simulink model "untitled"  (R2022a)
settings: Solver=VariableStepAuto  StartTime=0.0  StopTime=6  RelTol=1e-3
libraries: spsSeriesRLCBranchLib x8, spsDiodeLib x6, spsVoltageMeasurementLib x4, spsACVoltageSourceLib x3, spsGroundLib x3, spsCurrentMeasurementLib x1, spsPermanentMagnetSynchronousMachineLib x1, spsThreePhaseVIMeasurementLib x1
settings Model: Creator=glopezc  LastModifiedBy=glopezc

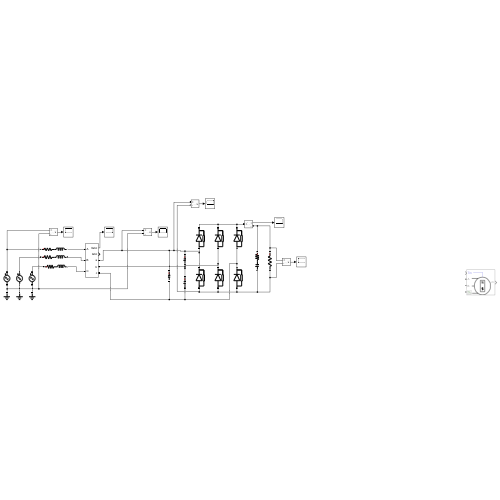
[thumbnail: Simulink's stored preview of the top-level diagram]
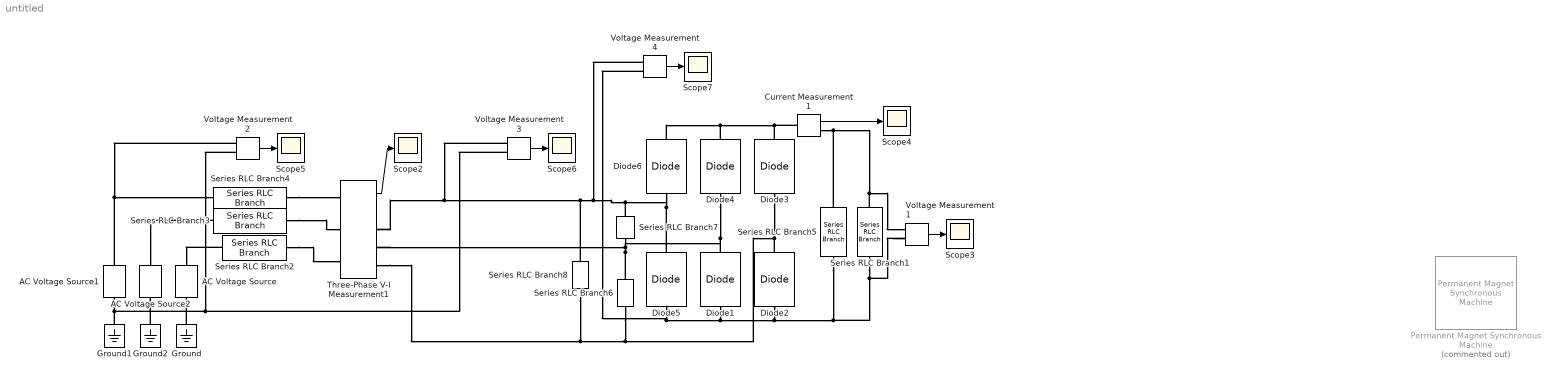
== system untitled ==
  AC Voltage Source : spsACVoltageSourceLib/AC Voltage Source  Amplitude=453  Phase=-120  Frequency=46  SampleTime=0  Measurements=None  BusType=swing  Pref=10e3  Qref=0  Qmin=-inf  Qmax=+inf
  AC Voltage Source1 : spsACVoltageSourceLib/AC Voltage Source  Amplitude=453  Phase=0  Frequency=46  SampleTime=0  Measurements=None  BusType=swing  Pref=10e3  Qref=0  Qmin=-inf  Qmax=+inf
  AC Voltage Source2 : spsACVoltageSourceLib/AC Voltage Source  Amplitude=453  Phase=120  Frequency=46  SampleTime=0  Measurements=None  BusType=swing  Pref=10e3  Qref=0  Qmin=-inf  Qmax=+inf
  Current Measurement1 : spsCurrentMeasurementLib/Current Measurement  PhasorSimulation=off  OutputType=Complex  PSBequivalent=0
  Diode{1..6} (6 alike) : spsDiodeLib/Diode  Ron=0.01  Lon=0  Vf=0.6  IC=0  UseSnubber=0  Rs=500  Cs=250e-9  Measurements=off
  Ground : spsGroundLib/Ground  LConnTagsString=a
  Ground1 : spsGroundLib/Ground  LConnTagsString=a
  Ground2 : spsGroundLib/Ground  LConnTagsString=a
  Permanent Magnet Synchronous Machine : spsPermanentMagnetSynchronousMachineLib/Permanent Magnet Synchronous Machine  Commented=on  NbPhases=3  FluxDistribution=Sinusoidal  RotorType=Round  MechanicalLoad=Torque Tm  PresetModel=No  ShowDetailedParameters=on  MeasurementBus=off  Resistance=0.0485  Inductance=8.5e-3  dqInductances=[8.5e-3,8.5e-3]  La=0.000395  MachineConstant=Flux linkage established by magnets (V.s)  Flux=0.1194  VoltageCst=86.6271  TorqueCst=0.7164  Flat=120  Mechanical=[0.0027 0.0004924 4 0]  PolePairs=4  InitialConditions=[0,0, 0,0]  InitialConditions5ph=[0 0 0 0 0 0]  RefAngle=90 degrees behind phase A axis (modified Park)  IterativeDiscreteModel=Trapezoidal non iterative  TsBlock=-1  TsPowergui=0
  Scope{2..7} (6 alike) : Scope
  Series RLC Branch1 : spsSeriesRLCBranchLib/Series RLC Branch  LConnTagsString=__new0  RConnTagsString=__new0  BranchType=R  Resistance=.022e3  Inductance=1e-3  SetiL0=off  InitialCurrent=0  Capacitance=1e-6  Setx0=off  InitialVoltage=0  Measurements=None
  Series RLC Branch2 : spsSeriesRLCBranchLib/Series RLC Branch  LConnTagsString=__new0  RConnTagsString=__new0  BranchType=RL  Resistance=.51  Inductance=12.8e-3  SetiL0=off  InitialCurrent=0  Capacitance=1e-6  Setx0=off  InitialVoltage=0  Measurements=None
  Series RLC Branch3 : spsSeriesRLCBranchLib/Series RLC Branch  LConnTagsString=__new0  RConnTagsString=__new0  BranchType=RL  Resistance=.51  Inductance=12.8e-3  SetiL0=off  InitialCurrent=0  Capacitance=1e-6  Setx0=off  InitialVoltage=0  Measurements=None
  Series RLC Branch4 : spsSeriesRLCBranchLib/Series RLC Branch  LConnTagsString=__new0  RConnTagsString=__new0  BranchType=RL  Resistance=.51  Inductance=12.8e-3  SetiL0=off  InitialCurrent=0  Capacitance=1e-6  Setx0=off  InitialVoltage=0  Measurements=None
  Series RLC Branch5 : spsSeriesRLCBranchLib/Series RLC Branch  LConnTagsString=__new0  RConnTagsString=__new0  BranchType=RC  Resistance=.00084  Inductance=1e-3  SetiL0=off  InitialCurrent=0  Capacitance=2200e-6  Setx0=off  InitialVoltage=0  Measurements=None
  Series RLC Branch6 : spsSeriesRLCBranchLib/Series RLC Branch  LConnTagsString=__new0  RConnTagsString=__new0  BranchType=C  Resistance=0.001  Inductance=1e-3  SetiL0=off  InitialCurrent=0  Capacitance=55e-6  Setx0=off  InitialVoltage=0  Measurements=None
  Series RLC Branch7 : spsSeriesRLCBranchLib/Series RLC Branch  LConnTagsString=__new0  RConnTagsString=__new0  BranchType=C  Resistance=0.001  Inductance=1e-3  SetiL0=off  InitialCurrent=0  Capacitance=55e-6  Setx0=off  InitialVoltage=0  Measurements=None
  Series RLC Branch8 : spsSeriesRLCBranchLib/Series RLC Branch  LConnTagsString=__new0  RConnTagsString=__new0  BranchType=C  Resistance=0.001  Inductance=1e-3  SetiL0=off  InitialCurrent=0  Capacitance=55e-6  Setx0=off  InitialVoltage=0  Measurements=None
  Three-Phase V-I Measurement1 : spsThreePhaseVIMeasurementLib/Three-Phase V-I Measurement  VoltageMeasurement=phase-to-ground  SetLabelV=off  LabelV=Vabc  Vpu=off  VpuLL=off  CurrentMeasurement=yes  SetLabelI=off  LabelI=Iabc  Ipu=off  Pbase=100e6  Vbase=500e3  OutputType=Complex  PhasorSimulation=off  PSBequivalent=0
  Voltage Measurement{1..4} (4 alike) : spsVoltageMeasurementLib/Voltage Measurement  PhasorSimulation=off  OutputType=Complex  PSBequivalent=0
  wires:
  Current Measurement1/1 -> Scope4/1
  Voltage Measurement1/1 -> Scope3/1
  Three-Phase V-I Measurement1/1 -> Scope2/1
  Voltage Measurement2/1 -> Scope5/1
  Voltage Measurement3/1 -> Scope6/1
  Voltage Measurement4/1 -> Scope7/1
  connections:
  Three-Phase V-I Measurement1/RConn3 -- Series RLC Branch6/RConn1 -- Diode3/LConn1 -- Diode2/RConn1 -- Series RLC Branch8/RConn1
  Series RLC Branch7/RConn1 -- Three-Phase V-I Measurement1/RConn2 -- Diode4/LConn1 -- Diode1/RConn1 -- Series RLC Branch6/LConn1
  Current Measurement1/LConn1 -- Diode3/RConn1 -- Diode6/RConn1 -- Diode4/RConn1
  Voltage Measurement3/LConn1 -- Three-Phase V-I Measurement1/RConn1 -- Series RLC Branch8/LConn1 -- Series RLC Branch7/LConn1 -- Diode5/RConn1 -- Diode6/LConn1 -- Voltage Measurement4/LConn1
  Ground2/LConn1 -- AC Voltage Source2/LConn1
  Ground/LConn1 -- AC Voltage Source/LConn1
  Ground1/LConn1 -- Voltage Measurement2/LConn2 -- Voltage Measurement3/LConn2 -- AC Voltage Source1/LConn1
  Series RLC Branch1/RConn1 -- Voltage Measurement4/LConn2 -- Diode5/LConn1 -- Diode1/LConn1 -- Diode2/LConn1 -- Series RLC Branch5/RConn1 -- Voltage Measurement1/LConn2
  Series RLC Branch1/LConn1 -- Series RLC Branch5/LConn1 -- Current Measurement1/RConn1 -- Voltage Measurement1/LConn1
  Series RLC Branch2/RConn1 -- Three-Phase V-I Measurement1/LConn3
  Series RLC Branch2/LConn1 -- AC Voltage Source/RConn1
  Series RLC Branch3/RConn1 -- Three-Phase V-I Measurement1/LConn2
  Series RLC Branch3/LConn1 -- AC Voltage Source2/RConn1
  Series RLC Branch4/RConn1 -- Three-Phase V-I Measurement1/LConn1
  AC Voltage Source1/RConn1 -- Series RLC Branch4/LConn1 -- Voltage Measurement2/LConn1
